simulink model "ball_balancing_omni3_multibody_cascade"  (R2026a)
settings: Solver=ode15s  StopTime=ballbotParams.simulation.stopTime  MaxStep=ballbotParams.simulation.maxStep  RelTol=ballbotParams.simulation.relativeTolerance
PreLoadFcn:
  | ballbotParams = ballbotParameters; ballbotParams.controller.minimumContactConfidence = 0.10;
undefined symbols (not defined in the file or in its folder): ballbotCascadeBalanceAllocate, ballbotDcMotorTorqueEnvelope, ballbotEstimatorInitialState, ballbotEstimatorUpdate, ballbotImuFromJoint, ballbotPoseFromJoint, ballbotVelocityErrorBody, ballbotWheelRateFromDisplacement, X, Y, Z
libraries: sm_lib x26, nesl_utility x23
(part 3 of 3)

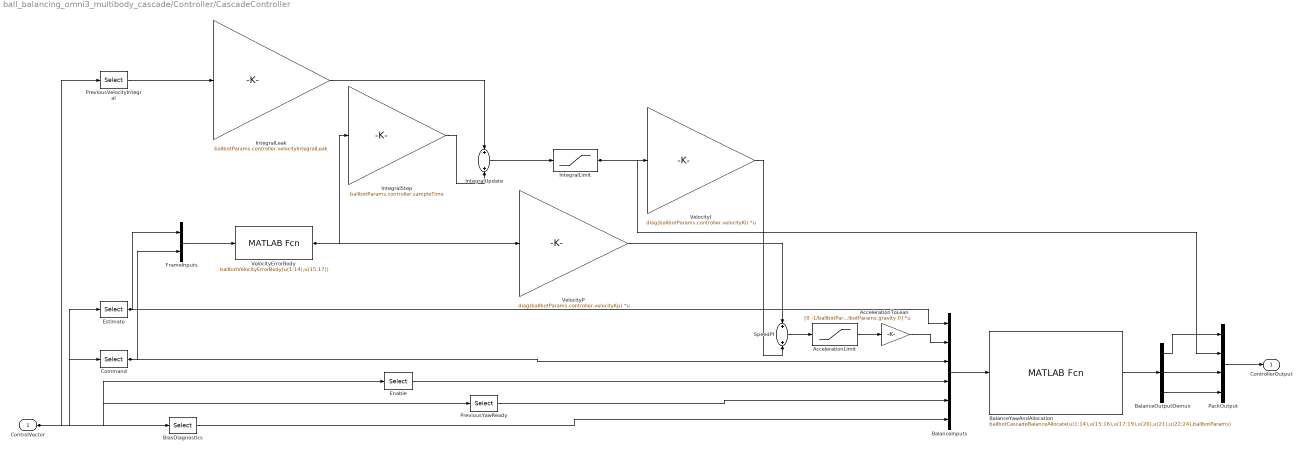
== system ball_balancing_omni3_multibody_cascade/Controller/CascadeController ==
  ControlVector : Inport
  AccelerationLimit : Saturate  UpperLimit=ballbotParams.controller.maxPlanarAcceleration  LowerLimit=-ballbotParams.controller.maxPlanarAcceleration
  AccelerationToLean : Gain  Gain=[0 -1/ballbotParams.gravity; 1/ballbotParams.gravity 0]  Multiplication=Matrix(K*u)
  BalanceInputs : Mux  Inputs=6
  BalanceOutputDemux : Demux  Outputs=[3 1 1]
  BalanceYawAndAllocation : MATLABFcn  MATLABFcn=ballbotCascadeBalanceAllocate(u(1:14),u(15:16),u(17:19),u(20),u(21),u(22:24),ballbotParams)  OutputDimensions=5  SampleTime=ballbotParams.controller.sampleTime
  BiasDiagnostics : Selector  InputPortWidth=24  IndexOptions=Index vector (dialog)  Indices=22:24  OutputSizes=1
  Command : Selector  InputPortWidth=24  IndexOptions=Index vector (dialog)  Indices=15:17  OutputSizes=1
  Enable : Selector  InputPortWidth=24  IndexOptions=Index vector (dialog)  Indices=20  OutputSizes=1
  Estimate : Selector  InputPortWidth=24  IndexOptions=Index vector (dialog)  Indices=1:14  OutputSizes=1
  FrameInputs : Mux  Inputs=2
  IntegralLeak : Gain  Gain=ballbotParams.controller.velocityIntegralLeak
  IntegralLimit : Saturate  UpperLimit=ballbotParams.controller.velocityIntegralLimit  LowerLimit=-ballbotParams.controller.velocityIntegralLimit
  IntegralStep : Gain  Gain=ballbotParams.controller.sampleTime
  IntegralUpdate : Sum
  PackOutput : Mux
  PreviousVelocityIntegral : Selector  InputPortWidth=24  IndexOptions=Index vector (dialog)  Indices=18:19  OutputSizes=1
  PreviousYawReady : Selector  InputPortWidth=24  IndexOptions=Index vector (dialog)  Indices=21  OutputSizes=1
  SpeedPI : Sum
  VelocityErrorBody : MATLABFcn  MATLABFcn=ballbotVelocityErrorBody(u(1:14),u(15:17))  OutputDimensions=2  SampleTime=ballbotParams.controller.sampleTime
  VelocityI : Gain  Gain=diag(ballbotParams.controller.velocityKi)  Multiplication=Matrix(K*u)
  VelocityP : Gain  Gain=diag(ballbotParams.controller.velocityKp)  Multiplication=Matrix(K*u)
  ControllerOutput : Outport
  wires:
  Estimate/1 -> BalanceInputs/1, FrameInputs/1
  ControlVector/1 -> Command/1, Estimate/1, PreviousYawReady/1, PreviousVelocityIntegral/1, BiasDiagnostics/1, Enable/1
  PreviousVelocityIntegral/1 -> IntegralLeak/1
  Command/1 -> BalanceInputs/3, FrameInputs/2
  VelocityErrorBody/1 -> VelocityP/1, IntegralStep/1
  FrameInputs/1 -> VelocityErrorBody/1
  IntegralLeak/1 -> IntegralUpdate/1
  BiasDiagnostics/1 -> BalanceInputs/6
  IntegralStep/1 -> IntegralUpdate/2
  Enable/1 -> BalanceInputs/4
  IntegralUpdate/1 -> IntegralLimit/1
  VelocityP/1 -> SpeedPI/1
  PreviousYawReady/1 -> BalanceInputs/5
  IntegralLimit/1 -> PackOutput/2, VelocityI/1
  VelocityI/1 -> SpeedPI/2
  SpeedPI/1 -> AccelerationLimit/1
  BalanceYawAndAllocation/1 -> BalanceOutputDemux/1
  AccelerationLimit/1 -> AccelerationToLean/1
  AccelerationToLean/1 -> BalanceInputs/2
  BalanceOutputDemux/3 -> PackOutput/4
  BalanceInputs/1 -> BalanceYawAndAllocation/1
  BalanceOutputDemux/1 -> PackOutput/1
  BalanceOutputDemux/2 -> PackOutput/3
  PackOutput/1 -> ControllerOutput/1
